simulink model "StandardPID"  (Simulink 7.8)
settings: Solver=ode45  StartTime=0.0  StopTime=10.0  RelTol=1e-3
settings Model: Creator=PC  LastModifiedBy=PC

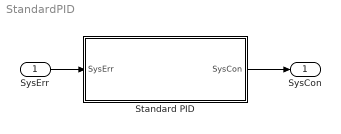
== system StandardPID ==
  SysErr : Inport
  Standard PID : Subsystem  mask{Kp=0, Ti=0, Td=0}
      mask prompts: Kp "Proportional Gain"; Ti "Integral Time-constant"; Td "Derivative Time-constant"
      mask help: u(s)=Kp*(1+1/sTi+sTd)
      mask Help: Sorry, no help information yet!
      mask Display:
      | disp(' Standard PID ');
      | port_label ('input',1,'e');
      | port_label ('output',1,'u')
  SysCon : Outport
  wires:
  SysErr/1 -> Standard PID/1(SysErr)
  Standard PID/1(SysCon) -> SysCon/1

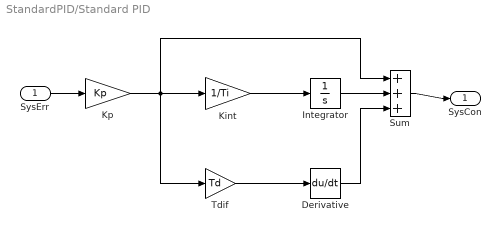
== system StandardPID/Standard PID ==
  SysErr : Inport
  Derivative : Derivative
  Integrator : Integrator
  Kint : Gain  Gain=1/Ti
  Kp : Gain  Gain=Kp
  Sum : Sum  Inputs=+++
  Tdif : Gain  Gain=Td
  SysCon : Outport
  wires:
  SysErr/1 -> Kp/1
  Kint/1 -> Integrator/1
  Integrator/1 -> Sum/2
  Sum/1 -> SysCon/1
  Derivative/1 -> Sum/3
  Tdif/1 -> Derivative/1
  Kp/1 -> Kint/1, Tdif/1, Sum/1
